simulink model "Samolot_simulink"  (R2021b)
settings: Solver=VariableStepAuto  StartTime=0.0  StopTime=10.0  RelTol=1e-3
undefined symbols (not defined in the file): h, k1, k2, m1, m2, m3, xdat, ydat
settings Model: Creator=revte  LastModifiedBy=revte

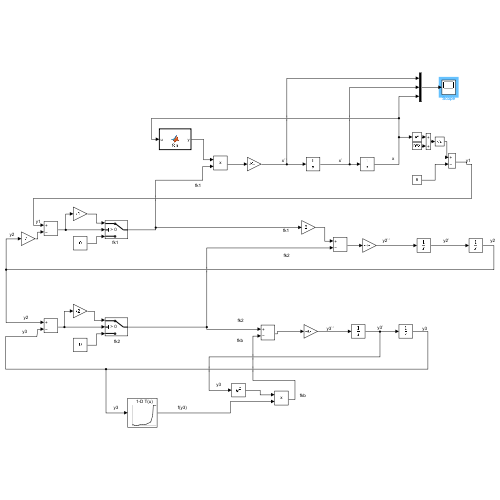
[thumbnail: Simulink's stored preview of the top-level diagram]
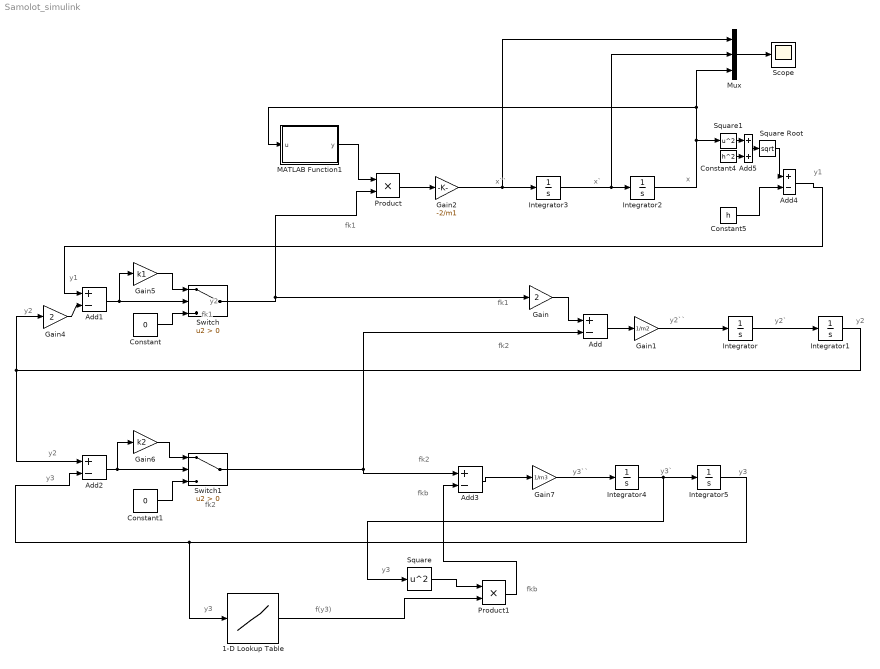
== system Samolot_simulink ==
  note: y3
  note: fkb
  note: y3
  note: f(y3)
  note: y3
  note: y3`
  note: y3``
  note: fkb
  note: fk2
  note: y3
  note: y2
  note: y2
  note: fk2
  note: fk1
  note: y2
  note: y1
  note: fk1
  note: x``
  note: x`
  note: x
  note: y2
  note: y2`
  note: y2``
  note: fk2
  note: fk1
  note: y1
  1-D Lookup Table : Lookup_n-D  NumberOfTableDimensions=1  BreakpointsForDimension1=xdat  Table=ydat  InternalRulePriority=Speed  RndMeth=Simplest  InputSameDT=on
  Add{,1..4} (5 alike) : Sum  Inputs=+-
  Add5 : Sum
  Constant : Constant  Value=0
  Constant1 : Constant  Value=0
  Constant4 : Constant  Value=h^2
  Constant5 : Constant  Value=h
  Gain : Gain  Gain=2
  Gain1 : Gain  Gain=1/m2
  Gain2 : Gain  Gain=-2/m1
  Gain4 : Gain  Gain=2
  Gain5 : Gain  Gain=k1
  Gain6 : Gain  Gain=k2
  Gain7 : Gain  Gain=1/m3
  Integrator{,1..2,4..5} (5 alike) : Integrator
  Integrator3 : Integrator  InitialCondition=67
  MATLAB Function1 : MATLAB Function  TreatAsAtomicUnit=on
  Mux : Mux  Inputs=3
  Product : Product
  Product1 : Product
  Scope : Scope
  Square : Math  Operator=square  SaturateOnIntegerOverflow=on
  Square Root : Sqrt  SaturateOnIntegerOverflow=on
  Square1 : Math  Operator=square  SaturateOnIntegerOverflow=on
  Switch : Switch  Criteria=u2 > Threshold
  Switch1 : Switch  Criteria=u2 > Threshold
  wires:
  Add4/1 -> Add1/1
  Gain/1 -> Add/1
  Switch1/1 -> Add3/1, Add/2
  Add/1 -> Gain1/1
  Gain1/1 -> Integrator/1
  Integrator/1 -> Integrator1/1
  Integrator1/1 -> Gain4/1, Add2/1
  Integrator2/1 -> Square1/1, Mux/3, MATLAB Function1/1(u)
  Integrator3/1 -> Mux/2, Integrator2/1
  Gain2/1 -> Mux/1, Integrator3/1
  Product/1 -> Gain2/1
  Switch/1 -> Product/2, Gain/1
  MATLAB Function1/1(y) -> Product/1
  Add1/1 -> Gain5/1, Switch/2
  Gain4/1 -> Add1/2
  Gain5/1 -> Switch/1
  Constant/1 -> Switch/3
  Constant1/1 -> Switch1/3
  Gain6/1 -> Switch1/1
  Add2/1 -> Gain6/1, Switch1/2
  Product1/1 -> Add3/2
  Add3/1 -> Gain7/1
  Gain7/1 -> Integrator4/1
  Integrator4/1 -> Square/1, Integrator5/1
  1-D Lookup Table/1 -> Product1/2
  Square/1 -> Product1/1
  Mux/1 -> Scope/1
  Constant5/1 -> Add4/2
  Square1/1 -> Add5/1
  Constant4/1 -> Add5/2
  Add5/1 -> Square Root/1
  Square Root/1 -> Add4/1
  Integrator5/1 -> 1-D Lookup Table/1, Add2/2

== matlab function Samolot_simulink/MATLAB Function1 ==
  data: u input; y output
function y = fcn(u)
h = 42;
y = u/sqrt(u^2+h^2);
